simulink model "PendulumModels"  (R2018b)
settings: Solver=ode4  StartTime=0.0  StopTime=20  FixedStep=10^-3  RelTol=1e-3
settings Model: Creator=Seko  LastModifiedBy=Seko

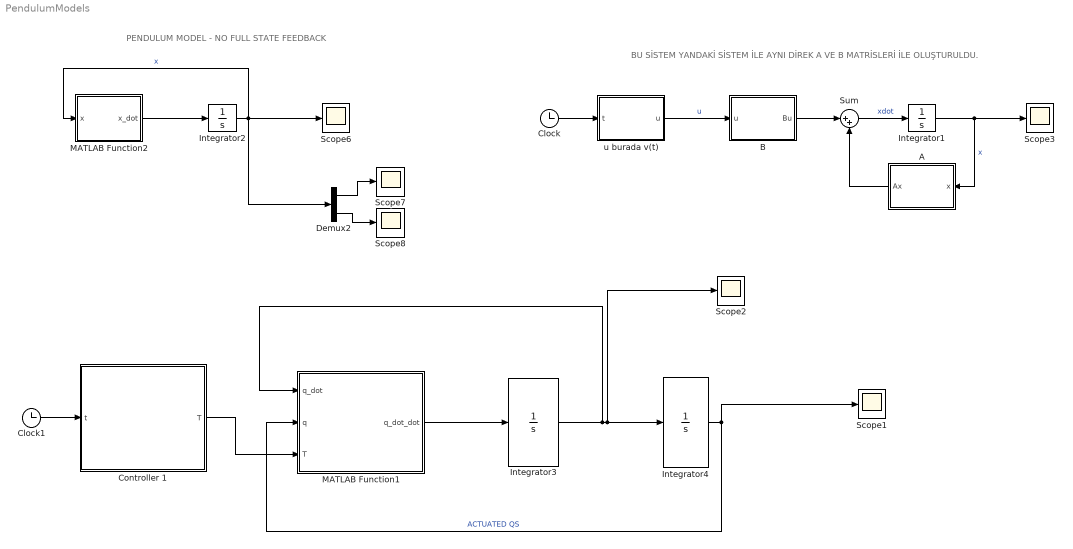
== system PendulumModels ==
  note: PENDULUM MODEL - NO FULL STATE FEEDBACK
  note: BU SİSTEM YANDAKİ SİSTEM İLE AYNI DİREK A VE B MATRİSLERİ İLE OLUŞTURULDU.
  A : MATLAB Function  TreatAsAtomicUnit=on
  B : MATLAB Function  TreatAsAtomicUnit=on
  Clock : Clock
  Clock1 : Clock
  Controller 1 : MATLAB Function  TreatAsAtomicUnit=on
  Demux2 : Demux  Outputs=2
  Integrator1 : Integrator  InitialCondition=[0;0]
  Integrator2 : Integrator  InitialCondition=[1;0]
  Integrator3 : Integrator  InitialCondition=[0]
  Integrator4 : Integrator  InitialCondition=[10]
  MATLAB Function1 : MATLAB Function  TreatAsAtomicUnit=on
  MATLAB Function2 : MATLAB Function  TreatAsAtomicUnit=on
  Scope{1..3,6..8} (6 alike) : Scope
  Sum : Sum  Inputs=|++
  "u burada v(t) " : MATLAB Function  TreatAsAtomicUnit=on
  wires:
  Integrator2/1 -> Demux2/1, Scope6/1, MATLAB Function2/1(x)  "x"
  MATLAB Function2/1(x_dot) -> Integrator2/1
  Demux2/1 -> Scope7/1
  Demux2/2 -> Scope8/1
  A/1(Ax) -> Sum/2
  B/1(Bu) -> Sum/1
  Sum/1 -> Integrator1/1  "xdot"
  Integrator1/1 -> Scope3/1, A/1(x)  "x"
  Clock/1 -> "u burada v(t) "/1(t)
  "u burada v(t) "/1(u) -> B/1(u)  "u"
  MATLAB Function1/1(q_dot_dot) -> Integrator3/1
  Integrator3/1 -> MATLAB Function1/1(q_dot), Scope2/1, Integrator4/1
  Integrator4/1 -> MATLAB Function1/2(q), Scope1/1  "ACTUATED QS"
  Clock1/1 -> Controller 1/1(t)
  Controller 1/1(T) -> MATLAB Function1/3(T)

== matlab function PendulumModels/MATLAB Function1 ==
  data: q_dot input; q_dot_dot output; q input; T input
function q_dot_dot = fcn(q_dot,q,T)

g=9.81;     %unit
m1=1.39355;
r1= 0.23678;
l1=  0.48373;
I1=0.07540282163;

Q1=q(1);   %RADYAN
Q1_DOT=q_dot(1); %RADYAN/S

b1=0.3;




alfa=I1+m1*r1^2;


M=[alfa]    

V=[b1*Q1_DOT]

G=[m1*g*r1*cos(Q1)] 

                                 
                                                                

q_dot_dot = (1/M)*(T-V-G);

end

== matlab function PendulumModels/Controller 1 ==
  data: t input; T output

function T  = fcn(t)


T=[0*t]

end

== matlab function PendulumModels/B ==
  data: u input; Bu output
function Bu = fcn(u)

%B matrisini tanımlıyoruz
%Real parameter values:
I=0.078; %[kg*m^2]
m=1.394; %[kg]
r=0.484; %[m]
g=9.8;   %[m/s^2]
b=0.5;   %damping coefficient

alfa=I+m*r^2;

b00=0;
b10=1/alfa;

B=[b00; 
   b10];
%B*x i tanımlıyoruz
Bu=B*u;

end

== matlab function PendulumModels/A ==
  data: x input; Ax output
function Ax = fcn(x)

%Real parameter values:
I=0.078; %[kg*m^2]
m=1.394; %[kg]
r=0.484; %[m]
g=9.8;   %[m/s^2]
b=5;   %damping coefficient

alfa=I+m*r^2;
beta=m*g*r;

%State space matrix (Bunu video 21'de çıkardık)
a00=0;
a01=1;
a10= -beta/alfa;
a11= b/alfa;

A=[a00,a01;
   a10,a11];
Ax= A*x;
end

== matlab function PendulumModels/MATLAB Function2 ==
  data: x input; x_dot output
function x_dot = fcn(x)
%% Pendulum sistemi için A ve B state space matrislerini oluşturulaım:


%Real parameter values:
I=0.078; %[kg*m^2]
m=1.394; %[kg]
r=0.484; %[m]
g=9.8;   %[m/s^2]
b=5;   %damping coefficient

alfa=I+m*r^2;
beta=m*g*r;

%State space matrix (Bunu video 21'de çıkardık)
a00=0;
a01=1;
a10= -beta/alfa;
a11= b/alfa;

b00=0;
b10=1/alfa;

A=[a00,a01;
   a10,a11];

B=[b00; 
    b10];
%%

%% Sistemin State Space Denklemi'ni yazıyoruz:
x_dot=A*x;

end

== matlab function PendulumModels/u burada v(t)  ==
  data: t input; u output
function u = fcn(t)
u=0*t;
end
